simulink model "uavPackageDelivery"  (R2024b)
settings: Solver=VariableStepAuto  StartTime=0.0  StopTime=simTime  FixedStep=.005  RelTol=1e-3  EnableMultiTasking=on
undefined symbols (not defined in the file): baseMission, Controller, DiscIntNeverNeededParam, Earth, Gravity, oaMission, startFlightTime, uavIC_latLon, UAVSampleTime, Vehicle, WGS84
libraries: slpidlib x4, uavalgslib x4, simulink x2, aerolibtransform2 x1, mspfiltlib x1, sharedTrackingLibrary x1
(part 2 of 2)

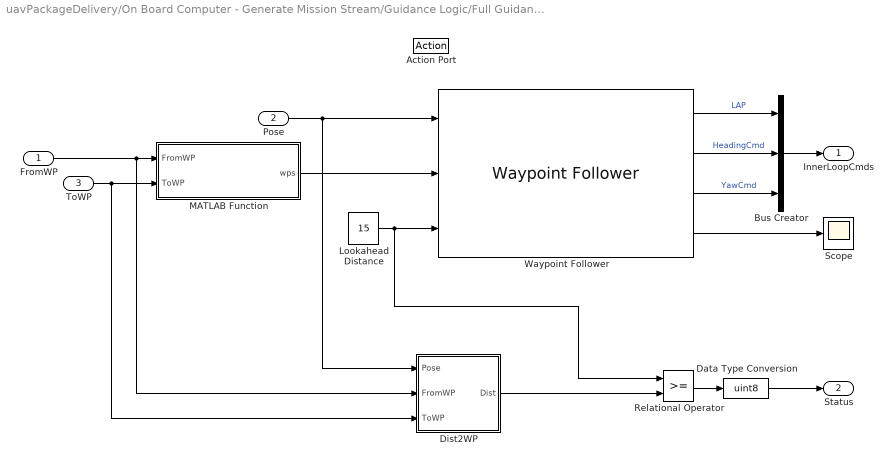
== system uavPackageDelivery/On Board Computer - Generate Mission Stream/Guidance Logic/Full Guidance Logic/Guidance Stateflow/Guidance Mode Selector/GuidanceLogic.WP ==
  FromWP : Inport
  Pose : Inport  Port=2
  ToWP : Inport  Port=3
  Action Port : ActionPort
      settings: CopyFcn=Stateflow.SLINSF.SimulinkMan.removeBlockPreDeleteFcn  PreDeleteFcn=Stateflow.SLINSF.SimulinkMan.unsafePredeleteFcn
  Bus Creator : BusCreator  Inputs=3  OutDataTypeStr=Bus: innerLoopCmdsBus  NonVirtualBus=on
  Data Type Conversion : DataTypeConversion  OutDataTypeStr=uint8  SaturateOnIntegerOverflow=off  RndMeth=Floor
  Dist2WP : Subsystem
  Lookahead Distance : Constant  Value=15  OutDataTypeStr=single
  MATLAB Function : MATLAB Function  TreatAsAtomicUnit=on
  Relational Operator : RelationalOperator  OutDataTypeStr=boolean  RndMeth=Simplest  InputSameDT=off
  Scope : Scope
  Waypoint Follower : uavalgslib/Waypoint Follower  UAVType=multirotor  StartFrom=closest  TransitionRadiusSource=internal  TransitionRadius=10  MinLookaheadDistance=0.1  HoverAtLastWaypoint=off  YawInput=on  ShowCrossTrackErrorOutput=off  ShowStatusOutput=off  SimulateUsing=Code generation
  InnerLoopCmds : Outport  OutDataTypeStr=Bus: innerLoopCmdsBus
  Status : Outport  Port=2
  wires:
  Data Type Conversion/1 -> Status/1
  Bus Creator/1 -> InnerLoopCmds/1
  ToWP/1 -> Dist2WP/3(ToWP), MATLAB Function/2(ToWP)
  Waypoint Follower/1 -> Bus Creator/1  "LAP"
  MATLAB Function/1(wps) -> Waypoint Follower/2
  Waypoint Follower/2 -> Bus Creator/2  "HeadingCmd"
  Waypoint Follower/3 -> Bus Creator/3  "YawCmd"
  Lookahead Distance/1 -> Relational Operator/1, Waypoint Follower/3
  Pose/1 -> Waypoint Follower/1, Dist2WP/1(Pose)
  Waypoint Follower/4 -> Scope/1
  Dist2WP/1(Dist) -> Relational Operator/2
  FromWP/1 -> Dist2WP/2(FromWP), MATLAB Function/1(FromWP)
  Relational Operator/1 -> Data Type Conversion/1

== system uavPackageDelivery/On Board Computer - Generate Mission Stream/Guidance Logic/Full Guidance Logic/Guidance Stateflow/Guidance Mode Selector/GuidanceLogic.WP/Dist2WP ==
  Pose : Inport
  FromWP : Inport  Port=2
  ToWP : Inport  Port=3
  Bus Selector : BusSelector  OutputSignals=position
  Bus Selector1 : BusSelector  OutputSignals=position
  Demux : Demux  Outputs=[3 1]
  Dot Product : DotProduct  OutDataTypeStr=Inherit: Inherit via internal rule
  Subsystem : Subsystem
  Sum : Sum  Inputs=|-+
  Sum1 : Sum  Inputs=|+-
  Terminator : Terminator
  Dist : Outport
  wires:
  Sum1/1 -> Subsystem/1(V)
  Demux/2 -> Terminator/1
  Bus Selector/1 -> Sum/2, Sum1/1  "<position>"
  Demux/1 -> Sum/1
  Bus Selector1/1 -> Sum1/2  "<position>"
  Sum/1 -> Dot Product/1
  Subsystem/1(V_unit) -> Dot Product/2
  Pose/1 -> Demux/1
  Dot Product/1 -> Dist/1
  ToWP/1 -> Bus Selector/1
  FromWP/1 -> Bus Selector1/1

== system uavPackageDelivery/On Board Computer - Generate Mission Stream/Guidance Logic/Full Guidance Logic/Guidance Stateflow/Guidance Mode Selector/GuidanceLogic.WP/Dist2WP/Subsystem ==
  V : Inport
  Dot Product1 : DotProduct  OutDataTypeStr=Inherit: Inherit via internal rule
  Product : Product  Inputs=*/
  Saturation : Saturate  UpperLimit=inf  LowerLimit=0.00001
  Sqrt : Sqrt
  V_unit : Outport
  wires:
  V/1 -> Dot Product1/2, Dot Product1/1, Product/1
  Sqrt/1 -> Product/2
  Dot Product1/1 -> Saturation/1
  Saturation/1 -> Sqrt/1
  Product/1 -> V_unit/1

== matlab function uavPackageDelivery/On Board Computer - Data Fusion/ProcessSensorData/Show Camera Image ==
  data: imageFrame input
function plotImageFrame(imageFrame)

coder.extrinsic('ishandle','image');

persistent fig;

if isempty(fig)
    fig = figure();
    ax = newplot(fig);
    title(ax, 'Front-facing camera');
end

if ~isempty(fig) && ishandle(fig)
    ax = newplot(fig);
    image(ax, imageFrame);
    axis(ax, 'off');
end

== matlab function uavPackageDelivery/On Board Computer - Control System/Control Loop/Control System/Controller/Position Controller/Velocity error transformation (Earth to Body frame) ==
  data: yaw input; xy_err_earth input; xy_err_body output
function xy_err_body = LTP2B2D(yaw,xy_err_earth)

transformation = [cos(yaw), sin(yaw); -sin(yaw),  cos(yaw)];
xy_err_body = transformation * xy_err_earth;


end

== matlab function uavPackageDelivery/On Board Computer - Generate Mission Stream/Guidance Logic/Full Guidance Logic/Guidance Stateflow/Guidance Mode Selector/GuidanceLogic.Land.ToLand/MATLAB Function ==
  data: FromWP input Bus: uavPathManagerBus size=1; wps output; ToWP input Bus: uavPathManagerBus size=1
function wps = getLandingWaypoint(FromWP, ToWP)

persistent outWPS

if isempty(outWPS)
    outWPS = single(zeros(2,4));
end

outWPS(1,:) = [FromWP.position' FromWP.params(4)];
outWPS(2,:) = [ToWP.position(1:2)' FromWP.position(3) ToWP.params(4)];

wps = outWPS;

== matlab function uavPackageDelivery/Ground Control Station/Get Flight Mission/QGC/Mission to Xe/MATLAB Function ==
  data: mission input Bus: uavPathManagerBus size=42; waypoints output single size=[42 3]
function waypoints  = buildUAVMission(mission)
%
waypoints = single(zeros(42,3));

for i=1:length(mission)
    waypoints(i,1:3) = mission(i).position;
end

end

== matlab function uavPackageDelivery/Ground Control Station/Get Flight Mission/QGC/Create Mission for Path Manager ==
  data: baseMission input Bus: uavPathManagerBus size=42; isNew input size=1; LTPMission input size=[42 3]; mission output Bus: uavPathManagerBus size=42; qgcMission input Bus: uavPathManagerBus size=42
function mission = generateWaypointStream(baseMission, isNew, LTPMission, qgcMission)

persistent UAVMission

if isempty(UAVMission)
    UAVMission = baseMission;
end

%% If we got a new mission
if (isNew == true)
   for ii=1:42
       if LTPMission(ii,2) < 7275326
           UAVMission(ii).position = LTPMission(ii,:)';
           y = isnan(qgcMission(ii).params);
           UAVMission(ii).params = qgcMission(ii).params;
           if sum(y)>0
               UAVMission(ii).params(y) = single(0);
           end
           UAVMission(ii).mode = mavlinkToPlannerType(qgcMission(ii).mode);
       end
   end
end

mission = UAVMission;

end

function plannerType =  mavlinkToPlannerType (mavlinkType)
% see enum name="MAV_CMD" in common.xml for values.
    switch mavlinkType
        case 16 %MAV_CMD_NAV_WAYPOINT
            plannerType = uint8(2);
        case 18 %MAV_CMD_NAV_LOITER_TURNS
            plannerType = uint8(3);
        case 21 %MAV_CMD_NAV_LAND
            plannerType = uint8(4);
        case 22 %MAV_CMD_NAV_TAKEOFF
            plannerType = uint8(1);
        otherwise %this will likely error out to signal something unexpected
            plannerType = uint8(0);
    end
end

== matlab function uavPackageDelivery/On Board Computer - Generate Mission Stream/Guidance Logic/Full Guidance Logic/Guidance Stateflow/Guidance Mode Selector/GuidanceLogic.WP/MATLAB Function ==
  data: FromWP input Bus: uavPathManagerBus size=1; wps output; ToWP input Bus: uavPathManagerBus size=1
function wps = getWaypointMission(FromWP, ToWP)

persistent outWPS

if isempty(outWPS)
    outWPS = single(zeros(2,4));
end

outWPS(1,:) = [FromWP.position' FromWP.params(4)];
outWPS(2,:) = [ToWP.position' ToWP.params(4)];

% for ii=1:2
%     outWPS(ii,1:3) = GCSMission(ii).position';
%     outWPS(ii,4) = GCSMission(ii).params(4);
% end

wps = outWPS;

== matlab function uavPackageDelivery/On Board Computer - Control System/Control Loop/Control System/Controller/Yaw Controller/MATLAB Function ==
  data: u input; y output
function y = wrapYaw(u)
%u error in rad in -2pi to 2pi

if (u>pi)
    y = u-2*pi;
elseif(u<-pi)
    y = u +2*pi;
else
    y=u;
end

== matlab function uavPackageDelivery/On Board Computer - Control System/Control Loop/Control System/Controller/Yaw Controller/MATLAB Function1 ==
  data: u input; y output
function y = wrapYaw(u)
%u error in rad in -2pi to 2pi

if (u>pi)
    y = u-2*pi;
elseif(u<-pi)
    y = u +2*pi;
else
    y=u;
end

== matlab function uavPackageDelivery/On Board Computer - Control System/Control Loop/Control System/Controller/Position Controller/Position error transformation (Earth to Body frame) ==
  data: yaw input; xy_err_earth input; xy_err_body output
function xy_err_body = LTP2B2D(yaw,xy_err_earth)

transformation = [cos(yaw), sin(yaw); -sin(yaw),  cos(yaw)];
xy_err_body = transformation * xy_err_earth;


end

== stateflow chart uavPackageDelivery/On Board Computer - Generate Mission Stream/Guidance Logic/Full Guidance Logic/Guidance Stateflow/Guidance Mode Selector ==
  settings: updateMethod=DISCRETE  sampleTime=UAVSampleTime*4
  state GuidanceLogic
    state OnGround
    state Takeoff
    state WP
    state Orbit
    state Land
      state ToLand
      state Descend
      (default) -> ToLand
      ToLand -> Descend : [norm(Pose(1:2)-ToWP.position(1:2)) <= 5]
    (default) -> OnGround
    OnGround -> (junction 5) : [startFlight==1]
    Takeoff -> WP : [Pose(3) <= ToWP.position(3)]{Status = 1;}
    GuidanceLogic -> (junction 5) : [hasChanged(mode)]
    (junction 5) -> Takeoff [order 1] : [mode == 1]
    (junction 5) -> (junction 12) [order 2]
    (junction 12) -> WP [order 1] : [mode==2]
    (junction 12) -> (junction 17) [order 2]
    (junction 17) -> Orbit [order 1] : [mode==3]
    (junction 17) -> (junction 22) [order 2]
    (junction 22) -> Land
    Land -> GuidanceLogic : [Pose(3)>=-0.1]{Status = 2;}
  (default) -> GuidanceLogic
  data: sf_internal_action_state_placeholder_data local double size=1 =0; sf_internal_action_state_placeholder_data local double size=1 =0; sf_internal_action_state_placeholder_data local double size=1 =0; sf_internal_action_state_placeholder_data local double size=1 =0; sf_internal_action_state_placeholder_data local double size=1 =0; mode input; ToWP input Bus: uavPathManagerBus; InnerLoopCmds output Bus: innerLoopCmdsBus; Status output uint8; FromWP input Bus: uavPathManagerBus; Pose input; startFlight input; GdncMode output Enum: GdncModeType
